simulink model "untitled"  (R2017b)
settings: Solver=VariableStepAuto  StartTime=0.0  StopTime=10.0  RelTol=1e-3
values from neighbouring files (symbols this model uses):
  C1 = N*Kd + Kp    (= 1.88646026293)    [lead_lag_comp_def.m]
  C2 = N*Kp    (= 1.88648445063e-07)    [lead_lag_comp_def.m]
  C3 = 1    [lead_lag_comp_def.m]
  C4 = N    (= 148.271702233)    [lead_lag_comp_def.m]
settings Model: Creator=13660  LastModifiedBy=13660

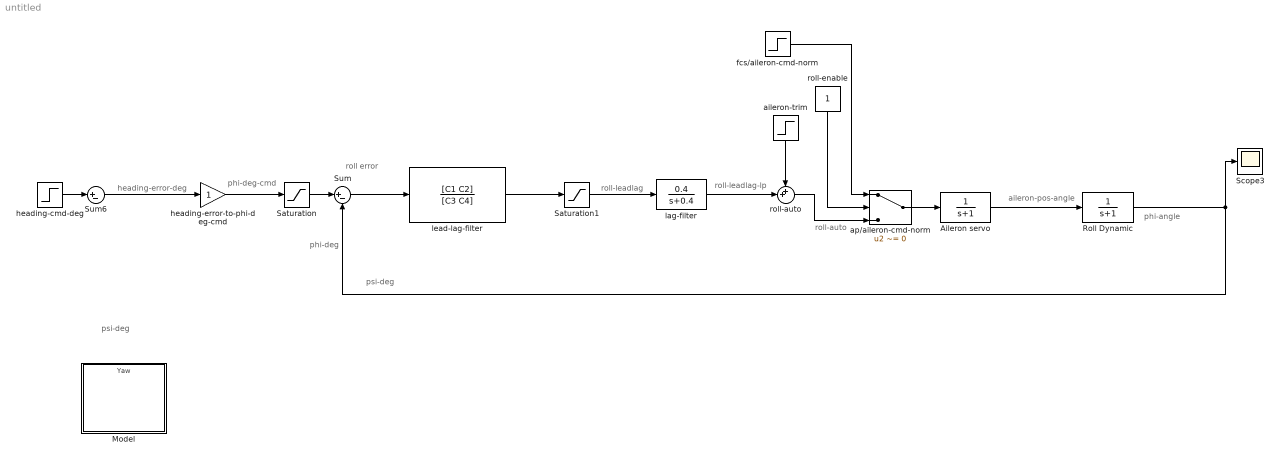
== system untitled ==
  note: psi-deg
  note: phi-angle
  note: aileron-pos-angle
  note: roll-auto
  note: roll-leadlag-lp
  note: roll-leadlag
  note: roll error
  note: phi-deg
  note: phi-deg-cmd
  note: heading-error-deg
  note: psi-deg
  Aileron servo : TransferFcn  Denominator=[1 1]
  Model : ModelReference  ModelNameDialog=Yaw.slx  SimulationMode=Normal  ModelReferenceVersion=1.1
  Roll Dynamic : TransferFcn  Denominator=[1 1]
  Saturation : Saturate  UpperLimit=30  LowerLimit=-30
  Saturation1 : Saturate  UpperLimit=0.1  LowerLimit=-0.1
  Scope3 : Scope
  Sum : Sum  Inputs=|+-
  Sum6 : Sum  Inputs=|+-
  aileron-trim : Step  SampleTime=0
  ap/aileron-cmd-norm : Switch  Criteria=u2 ~= 0
  fcs/aileron-cmd-norm : Step  SampleTime=0
  heading-cmd-deg : Step  SampleTime=0
  heading-error-to-phi-deg-cmd : Gain
  lag-filter : TransferFcn  Numerator=0.4  Denominator=[1 0.4]
  lead-lag-filter : TransferFcn  Numerator=[C1 C2]  Denominator=[C3 C4]
  roll-auto : Sum  Inputs=++|
  roll-enable : Constant
  wires:
  Sum6/1 -> heading-error-to-phi-deg-cmd/1
  lead-lag-filter/1 -> Saturation1/1
  heading-cmd-deg/1 -> Sum6/1
  heading-error-to-phi-deg-cmd/1 -> Saturation/1
  Saturation/1 -> Sum/1
  Roll Dynamic/1 -> Scope3/1, Sum/2
  Sum/1 -> lead-lag-filter/1
  Saturation1/1 -> lag-filter/1
  lag-filter/1 -> roll-auto/2
  aileron-trim/1 -> roll-auto/1
  roll-enable/1 -> ap/aileron-cmd-norm/2
  fcs/aileron-cmd-norm/1 -> ap/aileron-cmd-norm/1
  roll-auto/1 -> ap/aileron-cmd-norm/3
  ap/aileron-cmd-norm/1 -> Aileron servo/1
  Aileron servo/1 -> Roll Dynamic/1
  ? -> Sum6/2
